simulink model "simulink_model_pid_controller"  (R2022b)
settings: Solver=FixedStepAuto  StartTime=0.0  StopTime=1.0  RelTol=1e-3
undefined symbols (not defined in the file or in its folder): de_a, de_s, input
libraries: slpidlib x1
settings Model: Creator=giris  LastModifiedBy=giris

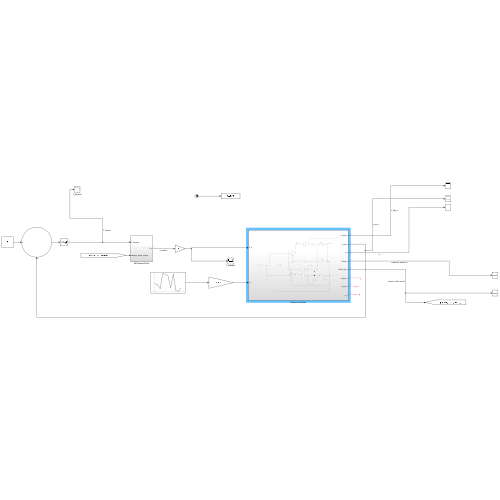
[thumbnail: Simulink's stored preview of the top-level diagram]
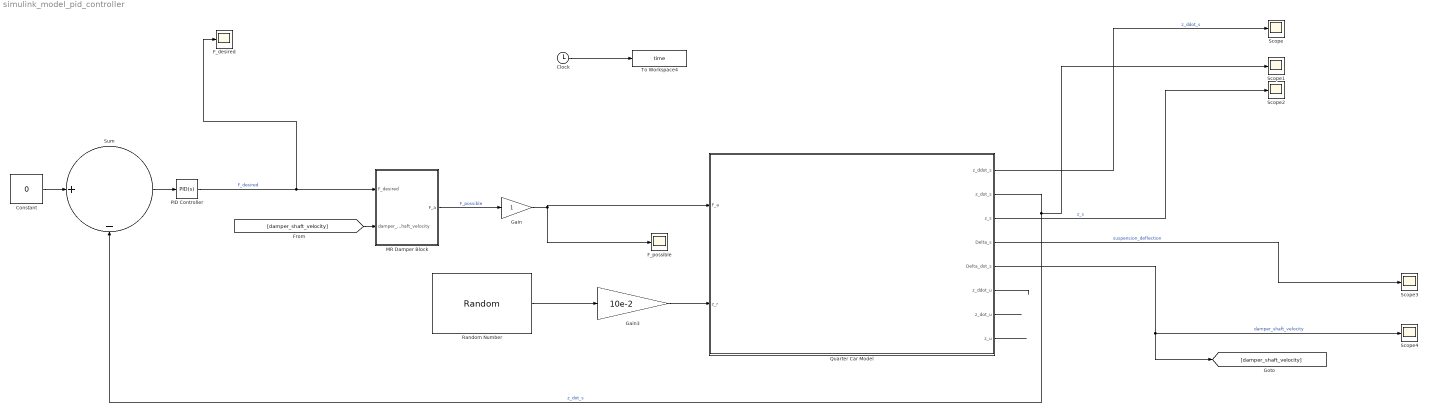
== system simulink_model_pid_controller ==
  Clock : Clock
      settings: Decimation=100
  Constant : Constant  Value=0
  F_desired : Scope
  F_possible : Scope
  Gain : Gain
  Gain3 : Gain  Gain=10e-2
  MR Damper Block : Subsystem
  PID Controller : slpidlib/PID Controller  Controller=PID  Form=Parallel  TimeDomain=Continuous-time  UseExternalTs=off  SampleTime=-1  IntegratorMethod=Forward Euler  FilterMethod=Forward Euler  ControllerParametersSource=internal  P=3500  I=100  UseKiTs=off  D=1000  N=100  UseFilter=on  TunerSelectOption=Transfer Function Based (PID Tuner App)  InitialConditionSource=internal  InitialConditionForIntegrator=0  InitialConditionForFilter=0  DifferentiatorICPrevScaledInput=0  ExternalReset=none  TrackingMode=off  Kt=1  LimitOutput=on  SatLimitsSource=internal  UpperSaturationLimit=inf  LowerSaturationLimit=-inf  LinearizeAsGain=on  AntiWindupMode=none  Kb=1  LimitIntegrator=off  UpperIntegratorSaturationLimit=inf  LowerIntegratorSaturationLimit=-inf  POutMin=[]  POutMax=[]  IOutMin=[]  IOutMax=[]  DOutMin=[]  DOutMax=[]  NOutMin=[]  NOutMax=[]  SumOutMin=[]  SumOutMax=[]  SaturationOutMin=[]  SaturationOutMax=[]  PParamMin=[]  PParamMax=[]  IParamMin=[]  IParamMax=[]  DParamMin=[]  DParamMax=[]  NParamMin=[]  NParamMax=[]  KbParamMin=[]  KbParamMax=[]  KtParamMin=[]  KtParamMax=[]  KbOutMin=[]  KbOutMax=[]  KtOutMin=[]  KtOutMax=[]  IntegratorOutMin=[]  IntegratorOutMax=[]  FilterOutMin=[]  FilterOutMax=[]  SumI1OutMin=[]  SumI1OutMax=[]  SumI2OutMin=[]  SumI2OutMax=[]  SumI3OutMin=[]  SumI3OutMax=[]  SumI4OutMin=[]  SumI4OutMax=[]  SumDOutMin=[]  SumDOutMax=[]  DifferentiatorOutMin=[]  DifferentiatorOutMax=[]  FilterDiffOutCoefMin=[]  FilterDiffOutCoefMax=[]  ReciprocalOutMin=[]  ReciprocalOutMax=[]  SumDenOutMin=[]  SumDenOutMax=[]  SumNumOutMin=[]  SumNumOutMax=[]  DivideOutMin=[]  DivideOutMax=[]  UdiffTsProdOutMin=[]  UdiffTsProdOutMax=[]  NTsProdOutMin=[]  NTsProdOutMax=[]  UintegralTsProdOutMin=[]  UintegralTsProdOutMax=[]  UngainTsProdOutMin=[]  UngainTsProdOutMax=[]  ClampingZeroOutDataTypeStr=Inherit: Inherit via back propagation  ClampingZeroOutMin=[]  ClampingZeroOutMax=[]  FilterDenConstantOutDataTypeStr=Inherit: Inherit via back propagation  FilterDenConstantOutMin=[]  FilterDenConstantOutMax=[]  PCopyOutDataTypeStr=Inherit: Inherit via back propagation  PCopyOutMin=[]  PCopyOutMax=[]  NCopyOutDataTypeStr=Inherit: Inherit via back propagation  NCopyOutMin=[]  NCopyOutMax=[]  IntegratorContinuousStateAttributes=''  IntegratorStateMustResolveToSignalObject=off  IntegratorRTWStateStorageClass=Auto  FilterContinuousStateAttributes=''  FilterStateMustResolveToSignalObject=off  FilterRTWStateStorageClass=Auto  ParallelPVariant=InternalParameters  IdealPVariant=Disabled  IVariant=InternalParameters  DVariant=InternalParameters  IntegratorVariant=Continuous  SatVariant=Disabled  AWVariant=Passthrough  PCopyVariant=Disabled  TRVariant=Disabled  FdbkBlocksVariant=Forward  IdealPFdbkVariant=Disabled  SatFdbkVariant=Disabled  DerivativeFilterVariant=ContFilter  NVariant=InternalParameters  NCopyVariant=Disabled  FilterICVariant=InternalICsFilter  IntegratorICVariant=InternalICs  ExternalResetVariant=Disabled  TRSumVariant=Passthrough  SumFdbkVariant=Disabled  SumVariant=Sum_PID  TsampFilterVariant=InternalTs  TsampNgainVariant=Passthrough  TsampIntegralVariant=Passthrough  ExternalSaturationOutDataTypeStr=Inherit: Same as second input
  Quarter Car Model : Subsystem
  Random Number : RandomNumber  SampleTime=0.001
  Scope{,1..4} (5 alike) : Scope
  Sum : Sum  Inputs=|+-
  To Workspace4 : ToWorkspace  VariableName=time  SampleTime=-1
  wires:
  Clock/1 -> To Workspace4/1
  Random Number/1 -> Gain3/1
  Gain3/1 -> Quarter Car Model/2(z_r)
  Quarter Car Model/1(z_ddot_s) -> Scope/1  "z_ddot_s"
  Quarter Car Model/2(z_dot_s) -> Sum/2, Scope1/1  "z_dot_s"
  Quarter Car Model/3(z_s) -> Scope2/1  "z_s"
  Quarter Car Model/4(Delta_s) -> Scope3/1  "suspension_deflection"
  Quarter Car Model/5(Delta_dot_s) -> [damper_shaft_velocity], Scope4/1  "damper_shaft_velocity"
  Constant/1 -> Sum/1
  Sum/1 -> PID Controller/1
  PID Controller/1 -> F_desired/1, MR Damper Block/1(F_desired)  "F_desired"
  [damper_shaft_velocity] -> MR Damper Block/2(damper_shaft_velocity)
  MR Damper Block/1(F_a) -> Gain/1  "F_possible"
  Gain/1 -> F_possible/1, Quarter Car Model/1(F_a)
  Quarter Car Model/6(z_ddot_u) -> ?
  Quarter Car Model/7(z_dot_u) -> ?
  Quarter Car Model/8(z_u) -> ?

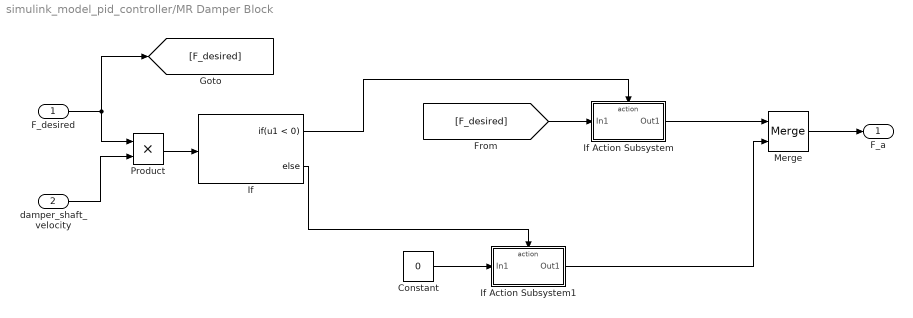
== system simulink_model_pid_controller/MR Damper Block ==
  F_desired : Inport
  damper_shaft_velocity : Inport  Port=2
  Constant : Constant  Value=0
  If : If  IfExpression=u1 < 0
  If Action Subsystem : Subsystem  TreatAsAtomicUnit=on
  If Action Subsystem1 : Subsystem  TreatAsAtomicUnit=on
  Merge : Merge
  Product : Product
  F_a : Outport
  wires:
  F_desired/1 -> [F_desired], Product/1
  damper_shaft_velocity/1 -> Product/2
  Product/1 -> If/1
  If/1 -> If Action Subsystem/Action
  If Action Subsystem/1(Out1) -> Merge/1
  If/2 -> If Action Subsystem1/Action
  Constant/1 -> If Action Subsystem1/1(In1)
  If Action Subsystem1/1(Out1) -> Merge/2
  Merge/1 -> F_a/1
  [F_desired] -> If Action Subsystem/1(In1)

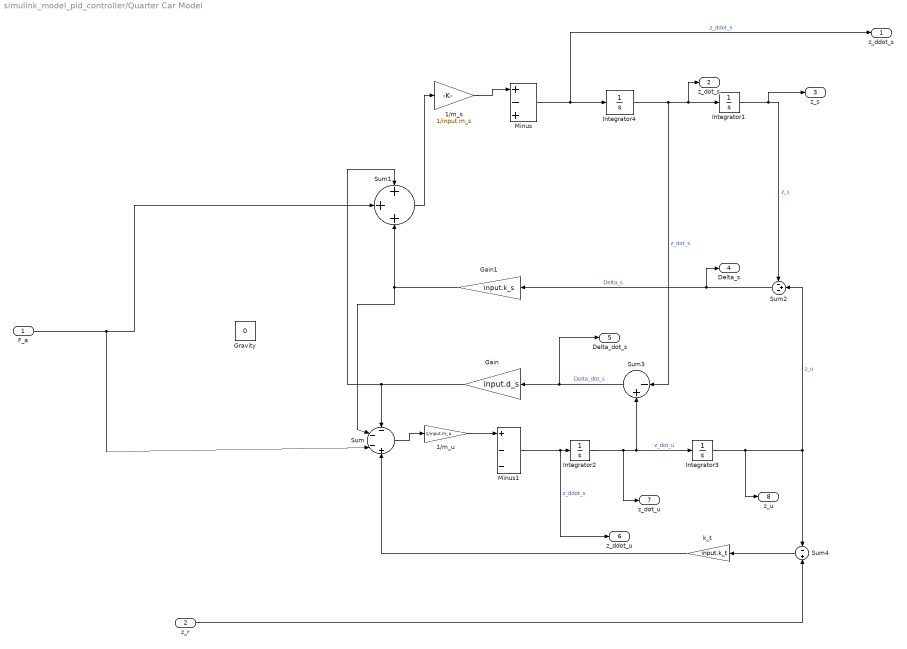
== system simulink_model_pid_controller/Quarter Car Model ==
  F_a : Inport
  z_r : Inport  Port=2
  1/m_s : Gain  Gain=1/input.m_s
  1/m_u : Gain  Gain=1/input.m_a
  Gain : Gain  Gain=input.d_s
  Gain1 : Gain  Gain=input.k_s
  Gravity : Constant  Value=0
  Integrator1 : Integrator  LowerSaturationLimit=de_s
  Integrator2 : Integrator
  Integrator3 : Integrator  LowerSaturationLimit=de_a
  Integrator4 : Integrator
  Minus : Sum  Inputs=+-+
  Minus1 : Sum  Inputs=+--
  Sum : Sum  Inputs=---+
  Sum1 : Sum  Inputs=+++
  Sum2 : Sum  Inputs=-+-
  Sum3 : Sum  Inputs=|-+
  Sum4 : Sum  Inputs=-+
  k_t : Gain  Gain=input.k_t
  z_ddot_s : Outport
  z_dot_s : Outport  Port=2
  z_s : Outport  Port=3
  Delta_s : Outport  Port=4
  Delta_dot_s : Outport  Port=5
  z_ddot_u : Outport  Port=6
  z_dot_u : Outport  Port=7
  z_u : Outport  Port=8
  wires:
  Sum1/1 -> 1/m_s/1
  Gain1/1 -> Sum1/3, Sum/2
  Sum4/1 -> k_t/1
  Integrator4/1 -> z_dot_s/1, Integrator1/1, Sum3/1  "z_dot_s"
  Minus1/1 -> z_ddot_u/1, Integrator2/1  "z_ddot_s"
  k_t/1 -> Sum/4
  Integrator1/1 -> z_s/1, Sum2/1  "z_s"
  1/m_s/1 -> Minus/1
  Sum2/1 -> Delta_s/1, Gain1/1  "Delta_s"
  Minus/1 -> z_ddot_s/1, Integrator4/1  "z_ddot_s"
  1/m_u/1 -> Minus1/1
  Gain/1 -> Sum1/1, Sum/1
  Integrator2/1 -> z_dot_u/1, Sum3/2, Integrator3/1  "z_dot_u"
  Integrator3/1 -> z_u/1, Sum2/2, Sum4/1  "z_u"
  Sum/1 -> 1/m_u/1
  Sum3/1 -> Delta_dot_s/1, Gain/1  "Delta_dot_s"
  z_r/1 -> Sum4/2
  F_a/1 -> Sum/3, Sum1/2

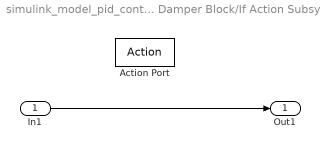
== system simulink_model_pid_controller/MR Damper Block/If Action Subsystem ==
  In1 : Inport
  Action Port : ActionPort  ActionPortLabel=if(u1 < 0)
  Out1 : Outport
  wires:
  In1/1 -> Out1/1

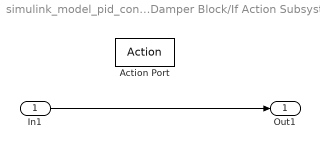
== system simulink_model_pid_controller/MR Damper Block/If Action Subsystem1 ==
  In1 : Inport
  Action Port : ActionPort  ActionPortLabel=else
  Out1 : Outport
  wires:
  In1/1 -> Out1/1
